simulink library "Library_SII_2018"  (R2018b)
settings: Solver=ode45  StartTime=0.0  StopTime=10.0  RelTol=1e-3  EnableMultiTasking=on
undefined symbols (not defined in the file or in its folder): coder, gcbh, r, simscape
libraries: fl_lib x157, nesl_utility x81, Library_SII2 x44, simulink x17, powerlib x12, mblibv1 x11, Simscape_SII_lib x11, elec_lib x10, Pneumatic_lib x4, $bdroot x2, peRmsMeasurement x1, powerlib_extras x1
(part 2 of 6)

== system Library_SII_2018/Mécanique ==
  Capteur de force FSR : Subsystem  mask(Capteur de force FSR){a=-0.8, b=5.2}
      mask help:
      | Modèle :
      | log(R) = a log(F) + b
      | avec :
      |   - F : force en N
      |   - R : résistance en Ohm
      mask DialogControl ParameterGroupVar Prompt: Paramètres
      mask Display: image('images/FSR.png')
  Capteur de puissance mécanique de rotation : Subsystem  mask(Capteur de puissance mécanique de rotation){}
      mask help:
      | Le bloc représente un capteur de puissance mécanique de rotation.
      | R et C sont des ports physiques conservatifs.
      |
      | P, T et W sont des ports Simulink délivrant les valeurs de :
      |  - la puissance mécanique traversant le bloc (en W)
      |  - le couple transmis à travers le bloc (en Nm)
      |  - la vitesse de rotation (en rad/s)
      |
      | Ces valeurs sont calculées par rapport au référentiel Ref.
      mask Display:
      | plot([149.600878633536;150.016472378793;150.47508104106;150.972287968219;151.50330478576;152.063017511447;152.646035805762;153.246744883819;153.859359588817;154.477980106257;155.096648782383;155.709407499646;156.310355056631;156.893703999851;157.453836360095;157.985357756531;158.483149347555;158.942417128023;159.358738098149;159.728102859405;160.046954227227;160.312221488639;160.521349974904;160.672325664379;160.763694578642;160.794576785101;160.764674871227;160.674276808796;160.524253180566;160.316048796087;160.051668777399;159.733659248606;159.365082815313;158.949489070056;158.490880407788;157.993673480629;157.462656663088;156.908284800231], [156.971389291536;157.430657072004;157.84697804213;158.216342803387;158.535194171208;158.80046143262;159.009589918885;159.16056560836;159.251934522623;159.282816729083;159.252914815208;159.162516752777;159.012493124547;158.804288740068;158.53990872138;158.221899192587;157.853322759294;157.437729014037;156.979120351769;156.48191342461;155.950896607069;155.391183881382;154.808165587067;154.20745650901;153.594841804012;152.976221286573;152.357552610446;151.744793893183;151.143846336199;150.560497392978;150.000365032735;149.468843636298;148.971052045274;148.511784264806;148.095463294681;147.726098533424;147.407247165603;147.144199990631])
      | plot([152.057635404444;152.93604260309;153.834625296826;154.744729643097;155.657590839533;156.564417533794;157.45647648909;158.325176690034;159.162152078811;159.959342124889;160.709069452336;161.404113777147;162.037781442523;162.603969882449;163.097226392739;163.512800643557;163.846690427691;164.095680203997;164.257372064819;164.330208829146;164.313489039122;164.27939575172], [142.228020686971;141.979030910664;141.817339049842;141.744502285515;141.761222075539;141.867337399197;142.061826307913;142.342815767178;142.707599694895;143.152665022428;143.673725527376;144.265763112236;144.923076131425;145.639334301243;146.40763966397;147.220593018964;148.070365181011;148.948772379657;149.847355073393;150.757459419663;151.6703206161;152.055850472277])
      | %plot([116.468514315784;116.438789536125;116.349901463023;116.202706137216;115.998621130155;115.739611892022;115.42817282337;115.067303252679;114.660478551187;114.211616663162;113.725040373958;113.205435679231;112.657806656235;112.087427271827;111.499790591278;110.900555877058;110.29549408704;109.690432297022;109.091197582803;108.503560902254;107.933181517846;107.38555249485;106.865947800123;106.379371510919;105.930509622894;105.523684921402;105.162815350711;104.851376282059;104.592367043926;104.388282036865;104.241086711057;104.152198637956;104.122473858297;104.152198637956;104.241086711057;104.388282036865;104.592367043926;104.851376282059;105.162815350711;105.523684921402;105.930509622894;106.379371510919;106.865947800123;107.38555249485;107.933181517846;108.503560902254;109.091197582803;109.690432297022;110.29549408704;110.900555877058;111.499790591278;112.087427271827;112.657806656235;113.205435679231;113.725040373958;114.211616663162;114.660478551187;115.067303252679;115.42817282337;115.739611892022;115.998621130155;116.202706137216;116.349901463023;116.438789536125;116.468514315784;116.468514315784], [111.618284136057;111.013222346039;110.413987631819;109.826350951271;109.255971566862;108.708342543866;108.188737849139;107.702161559936;107.253299671911;106.846474970419;106.485605399728;106.174166331075;105.915157092943;105.711072085881;105.563876760074;105.474988686973;105.445263907313;105.474988686973;105.563876760074;105.711072085881;105.915157092943;106.174166331075;106.485605399728;106.846474970419;107.253299671911;107.702161559936;108.188737849139;108.708342543866;109.255971566862;109.826350951271;110.413987631819;111.013222346039;111.618284136057;112.223345926075;112.822580640295;113.410217320843;113.980596705252;114.528225728247;115.047830422975;115.534406712178;115.983268600203;116.390093301695;116.750962872386;117.062401941038;117.321411179171;117.525496186232;117.67269151204;117.761579585141;117.7913043648;117.761579585141;117.67269151204;117.525496186232;117.321411179171;117.062401941038;116.750962872386;116.390093301695;115.983268600203;115.534406712178;115.047830422975;114.528225728247;113.980596705252;113.410217320843;112.822580640295;112.223345926075;111.618284136057;111.618284136057])
      | plot([239.23602886498;238.828071429858;237.608127977604;235.587947230552;232.78698463364;229.232214987837;224.957872668068;220.005121927465;214.421660463109;208.261260061133;201.583248745024;194.451939414329;186.936010476274;179.107844435155;171.042830809261;162.818640088593;154.514475725591;146.210311362589;137.986120641921;129.921107016027;122.092940974909;114.577012036853;107.445702706158;100.76769139005;94.607290988073;89.0238295237172;84.0710787831142;79.7967364633452;76.2419668175427;73.4410042206305;71.4208234735788;70.2008800213248;69.7929225862026;70.2008800213248;71.4208234735788;73.4410042206306;76.2419668175428;79.7967364633454;84.0710787831144;89.0238295237174;94.6072909880733;100.76769139005;107.445702706159;114.577012036853;122.092940974909;129.921107016027;137.986120641921;146.210311362589;154.514475725591;162.818640088593;171.042830809261;179.107844435155;186.936010476274;194.451939414329;201.583248745024;208.261260061133;214.421660463109;220.005121927465;224.957872668068;229.232214987837;232.78698463364;235.587947230552;237.608127977604;238.828071429858;239.23602886498;239.23602886498], [155.774275772274;147.47628550917;139.258209428443;131.199192095207;123.376846251889;115.866505365088;108.740498123116;102.067451871182;95.9116316925529;90.3323215006612;85.3832531026163;81.1120887325275;77.5599620381344;74.7610819412943;72.742403187363;71.5233667562631;71.1157126352191;71.5233667562631;72.742403187363;74.7610819412943;77.5599620381345;81.1120887325275;85.3832531026164;90.3323215006612;95.9116316925529;102.067451871182;108.740498123116;115.866505365089;123.376846251889;131.199192095207;139.258209428443;147.47628550917;155.774275772274;164.072266035377;172.290342116104;180.34935944934;188.171705292658;195.682046179459;202.808053421432;209.481099673365;215.636919851994;221.216230043886;226.165298441931;230.43646281202;233.988589506413;236.787469603253;238.806148357184;240.025184788284;240.432838909328;240.025184788284;238.806148357184;236.787469603253;233.988589506413;230.43646281202;226.165298441931;221.216230043886;215.636919851994;209.481099673365;202.808053421432;195.682046179459;188.171705292658;180.34935944934;172.290342116105;164.072266035378;155.774275772274;155.774275772274])
      | plot([252.715889364481;252.243022716633;250.828976737403;248.487369462568;245.240751850236;241.120390602797;236.165967051481;230.425195003451;223.953361231755;216.812793033479;209.072257983804;200.806301666664;192.094529760025;183.020841389688;173.672621134841;164.139897466795;154.514475725591;144.889053984387;135.356330316341;126.008110061494;116.934421691157;108.222649784518;99.9566934673787;92.2161584177032;85.075590219427;78.6037564477313;72.8629843997015;67.9085608483856;63.7881996009461;60.5415819886144;58.199974713779;56.7859287345493;56.3130620867014;56.7859287345493;58.1999747137791;60.5415819886146;63.7881996009463;67.9085608483858;72.8629843997018;78.6037564477315;85.0755902194273;92.2161584177035;99.9566934673791;108.222649784519;116.934421691157;126.008110061494;135.356330316341;144.889053984387;154.514475725591;164.139897466796;173.672621134841;183.020841389688;192.094529760025;200.806301666664;209.072257983803;216.812793033479;223.953361231755;230.425195003451;236.165967051481;241.120390602797;245.240751850236;248.487369462568;250.828976737403;252.243022716633;252.715889364481;252.715889364481], [154.514475725591;144.895228084285;135.36861905618;126.026395093992;116.958526921455;108.252343066071;99.9916888376535;92.2561188521535;85.1201308772245;78.6524483779929;72.9153586725213;67.9641130708855;63.8463947748555;60.6018596625959;58.2617543808809;56.8486154228053;56.3760520890355;56.8486154228053;58.2617543808809;60.6018596625959;63.8463947748555;67.9641130708856;72.9153586725213;78.652448377993;85.1201308772246;92.2561188521536;99.9916888376536;108.252343066072;116.958526921455;126.026395093992;135.36861905618;144.895228084285;154.514475725591;164.133723366898;173.660332395002;183.002556357191;192.070424529728;200.776608385111;209.037262613529;216.772832599029;223.908820573958;230.37650307319;236.113592778661;241.064838380297;245.182556676327;248.427091788587;250.767197070302;252.180336028377;252.652899362147;252.180336028377;250.767197070301;248.427091788587;245.182556676327;241.064838380297;236.113592778661;230.37650307319;223.908820573958;216.772832599029;209.037262613529;200.776608385111;192.070424529728;183.002556357191;173.660332395002;164.133723366898;154.514475725592;154.514475725591])
      | plot([154.514475725591;129.948374815285;179.017586633563;154.514475725591], [240.369848906994;203.583687543869;203.583687543869;240.369848906994])
      | %plot([105.382273904979;149.60125554353], [115.271704271436;156.971085816622])
      | plot([144.688035361469;144.688035361469], [152.057865634561;203.583687543869])
      | plot([164.277926087379;164.277926087379], [152.057865634561;203.583687543869])
      | plot([159.112745895982;159.616665914655], [149.60125554353;149.60125554353])
      | %plot([115.208714269102;159.364705905318], [107.901873998344;149.60125554353])
      | plot([0;311.800511553884;311.800511553884;0;0], [311.800511553884;311.800511553884;0;0;311.800511553884])
      | ;
      | color('red');
      | port_label('LConn', 1,'R')
      | port_label('RConn', 1,'C')
      | port_label('LConn', 2,'Ref')
      | port_label('output', 1,'P')
      | port_label('output', 2,'T')
      | port_label('output', 3,'W')
      | %port_label('RConn', 3,'A')
  Codeur incrémental : Subsystem  AncestorBlock=Library_SII/Signaux/Codeur incrémental  mask(Codeur incrémental bidirectionnel){p=1}
      mask prompts: p "Résolution du codeur [°]"
      mask help:
      | Codeur incrémental (linéaire ou rotatif)
      | En entrée : un signal analogique (quelle que soit la grandeur)
      | En sortie : deux signaux logiques de fréquence variable
      | Paramètre : pas du codeur (même grandeur que le signal d'entrée
      mask DialogControl ParameterGroupVar Prompt: Paramètre
      mask Display: image('codeur.png')
  Codeur incrémental v2 : Subsystem  AncestorBlock=Library_SII/Mécanique/Codeur incrémental  mask(Codeur incrémental bidirectionnel){p=1, U=5}
      mask prompts: p "Résolution du codeur [°]"; U "Amplitude des signaux"
      mask help:
      | Codeur incrémental (linéaire ou rotatif)
      | En entrée : un signal analogique (quelle que soit la grandeur)
      | En sortie : deux signaux logiques de fréquence variable
      | Paramètre : pas du codeur (même grandeur que le signal d'entrée
      mask DialogControl ParameterGroupVar Prompt: Paramètre
      mask Display: image('codeur.png')
  Corde : Subsystem  mask{L=0.2, S=1, E=210}
      mask prompts: L "Longueur [m]"; S "Section [mm²]"; E "Module d'élasticité [GPa]"
  Differentiel : Simscape_SII_lib/Differentiel  t_in_specify=off  t_in_priority=High  t_in=0 N*m  t_in_nominal_specify=off  t_in_nominal_unit=N*m  t_in_nominal_value=1  t_outG_specify=off  t_outG_priority=High  t_outG=0 N*m  t_outG_nominal_specify=off  t_outG_nominal_unit=N*m  t_outG_nominal_value=1  t_outD_specify=off  t_outD_priority=High  t_outD=0 N*m  t_outD_nominal_specify=off  t_outD_nominal_unit=N*m  t_outD_nominal_value=1
  Embrayage : Simscape_SII_lib/Embrayage  brkwy_trq=25 N*m  Col_trq=20 N*m  trans_coef=10 s/rad  vel_thr=1e-4 rad/s  w_specify=off  w_priority=High  w=0 rad/s  w_nominal_specify=off  w_nominal_unit=rad/s  w_nominal_value=1  t_specify=off  t_priority=High  t=0 N*m  t_nominal_specify=off  t_nominal_unit=N*m  t_nominal_value=1
  Embrayage SM : Subsystem  mask(Embrayage){axe=[0 0 1]}
      mask prompts: axe "Axe de la  liaison [x y z]"
      mask help:
      | Embrayage, basé sur une liaison pivot.
      |   C = Signal Simulink de commande
      |     C > 0 : état embrayé (transmission intégralle de la puissance)
      |     C = 0 : état débrayé (équivalent à une liaison pivot)
      |
      | Indiquer l'axe de la liaison par ses composantes dans World.
      mask Display:
      | image(imread('Mécanique/embrayage.png'))
      | port_label('lconn', 1, 'B')
      | port_label('rconn', 1, 'F')
      | port_label('input', 1, 'C')
  Engrenage droit SS : Subsystem  mask(Réducteur à engrenages droit){r=2, n=0.8, J=0.001}
      mask prompts: r "Rapport de transmission"; n "Rendement"; J "Inertie (kg/m^2)"
      mask help:
      | Réducteur à engrenages droit
      | P = Pignon
      | R = Roue
      | Ref = Référence
      |
      | Le rapport de réduction est défini par : wp/wr
      | Le rendement doit être compris entre 0.1 et 1
      mask Callback n:
      | ren = str2num(get_param(gcb,'n'));
      | if or((ren < 0.1),(ren > 1));
      |     errordlg('Le rendement doit etre compris entre 0.1 et 1','Erreur');
      | end;
      mask Display:
      | plot([0] , [0]);
      | 
      | color('red');
      | plot([30, 100] , [150, 150]);
      | plot([90, 110] , [180, 180]);
      | plot([90, 110] , [120, 120]);
      | plot([100, 100] , [120, 180]);
      | 
      | color('blue');
      | plot([100, 180] , [50, 50]);
      | plot([100, 100] , [0, 120]);
      | plot([90, 110] , [0, 0]);
      | 
      | color('black');
      | %image(imread('RoueVisSSFin.jpg'))
      | port_label('lconn', 1, 'P');
      | port_label('lconn', 2, 'Ref');
      | port_label('rconn', 1, 'R');
  Frein à courant de Foucault : Simscape_SII_lib/Frein à courant de Foucault  B=1 T  s=1 / 3.8e-8 S/m  e=3e-3 m  ra=20e-3 m  rd=120e-38 m  w_specify=off  w_priority=None  w=0 rad/s  w_nominal_specify=off  w_nominal_unit=rad/s  w_nominal_value=1  t_specify=off  t_priority=None  t=0 N*m  t_nominal_specify=off  t_nominal_unit=N*m  t_nominal_value=1
  Masse variable : Simscape_SII_lib/Masse variable  v_specify=off  v_priority=High  v=0 m/s  v_nominal_specify=off  v_nominal_unit=m/s  v_nominal_value=1  f_specify=off  f_priority=High  f=0 N  f_nominal_specify=off  f_nominal_unit=N  f_nominal_value=1
  Ressort lineaire (raideur variable) : Simscape_SII_lib/Ressort lineaire (raideur variable)  v_specify=off  v_priority=High  v=0 m/s  v_nominal_specify=off  v_nominal_unit=m/s  v_nominal_value=1  f_specify=off  f_priority=High  f=0 N  f_nominal_specify=off  f_nominal_unit=N  f_nominal_value=1  x_specify=off  x_priority=High  x=0 m  x_nominal_specify=off  x_nominal_unit=m  x_nominal_value=1
  Roue - Vis sans fin SS : Subsystem  mask(Engrenage à Roue et Vis sans fin){r=5, f=0.15, J=0.01, B=60}
      mask prompts: r "Rapport de transmission"; f "Coefficient de frottement"; J "Inertie (kg/m^2)"; B "Angle de denture  de la roue (°)"
      mask help:
      | Engrenage à Roue et Vis sans fin :
      | R = Roue
      | V = Vis
      | Ref = Référence
      |
      | Le rapport de transmission est défini par : r = Wv/Wr
      |
      | Les valeurs de l'angle de denture de la roue
      | et du coefficient de frottement
      | permettent de calculer le rendement (voir l'aide pour plus d'informations)
      | Selon que la vis ou la roue soit motrice, ce rendement varie
      | et l'on peut avoir irréversibilité.
      mask init:
      | % Angle de frottement (en rad)
      | P = atan(f);
      | 
      | % Angle de denture (en rad)
      | Br = pi*B/180;
      | 
      | % Rendements selon le sens
      | n1 = tan(Br)/tan(Br+P);
      | n2 = tan(Br-P)/tan(Br);
      mask Help:
      | Le rendement est calculé, selon le sens, par les expressions :
      |  - Vis motrice : n1 = tan(B)/tan(B+P)
      |  - Roue motrice : n2 = tan(B-P)/tan(B)
      | 
      | avec P = atan(f) : Angle de frottement
      mask Callback B:
      | if ( str2num(get_param(gcb, 'B')) <= 0);
      |      errordlg('L''angle de denture ne peut pas être négatif !','Erreur');
      | end;
      mask Display:
      | image(imread('Mécanique/RoueVisSSFin.jpg'));
      | port_label('lconn', 1, 'V');
      | port_label('lconn', 2, 'Ref');
      | port_label('rconn', 1, 'R');
  Roue libre SM : Subsystem  mask(Roue libre){axe=[1 0 0], kv=0.01}
      mask prompts: axe "Vecteur directeur [x y z]"; kv "Coefficient de frottement visqueux (Nm/(rad/s))"
      mask help:
      | Roue libre, basée sur une liaison pivot, mais la rotation n'est possible
      | que dans un seul sens.
      | Pour inverser le sens, inverser les connections B et F.
      |
      | Indiquer l'axe de la liaison par ses composantes dans World.
      mask Display:
      | image(imread('Mécanique/Roue_libre.png'))
      | port_label('lconn', 1, 'B')
      | port_label('rconn', 1, 'F')
  Réducteur avec rendement : Simscape_SII_lib/Réducteur avec rendement  rapport_transmission=10  rendement=0.8  t_in_specify=off  t_in_priority=High  t_in=0 N*m  t_in_nominal_specify=off  t_in_nominal_unit=N*m  t_in_nominal_value=1  t_out_specify=off  t_out_priority=High  t_out=0 N*m  t_out_nominal_specify=off  t_out_nominal_unit=N*m  t_out_nominal_value=1
  Réducteur avec rendement et frottement : Simscape_SII_lib/Réducteur avec rendement et frottement  rapport_transmission=10  rendement=0.8  Col_trq=1 N*m  t_in_specify=off  t_in_priority=None  t_in=0 N*m  t_in_nominal_specify=off  t_in_nominal_unit=N*m  t_in_nominal_value=1  t_out_specify=off  t_out_priority=None  t_out=0 N*m  t_out_nominal_specify=off  t_out_nominal_unit=N*m  t_out_nominal_value=1
  Train epicycloidal : Simscape_SII_lib/Train epicycloidal  ratio=2  t_R_specify=off  t_R_priority=High  t_R=0 N*m  t_R_nominal_specify=off  t_R_nominal_unit=N*m  t_R_nominal_value=1  t_S_specify=off  t_S_priority=High  t_S=0 N*m  t_S_nominal_specify=off  t_S_nominal_unit=N*m  t_S_nominal_value=1  t_C_specify=off  t_C_priority=High  t_C=0 N*m  t_C_nominal_specify=off  t_C_nominal_unit=N*m  t_C_nominal_value=1

== system Library_SII_2018/Signaux ==
  Codeur incrémental : Subsystem  mask(Codeur incrémental bidirectionnel){p=r}
      mask prompts: p "Pas du codeur"
      mask help:
      | Codeur incrémental (linéaire ou rotatif)
      | En entrée : un signal analogique (quelle que soit la grandeur)
      | En sortie : deux signaux logiques de fréquence variable
      | Paramètre : pas du codeur (même grandeur que le signal d'entrée
      mask DialogControl ParameterGroupVar Prompt: Paramètre
      mask Display: image('codeur.svg')
  Contrôle de régime : Subsystem  mask(Controleur de régime){vl=0.8, al=1}
      mask prompts: vl "Vitesse limite (1/s)"; al "Accélération limite (1/s²)"
      mask help:
      | Permet de limiter la vitesse et l'accélération de variation d'un signal
      | à partir d'un échelon.
      mask Callback al:
      | if str2num(get_param(gcb, 'vl'))<=0
      | 	error('La vitesse limite doit être strictement positive !')
      | end
      | if str2num(get_param(gcb, 'al'))<=0
      | 	error('L''accélération limite doit être strictement positive')
      | end
      mask Display:
      | color('red');
      | x = [10 15 20 25 30 35 40 45 55 60 65 70 75 80 85 90];
      | y = [10 10.68 12.72 16.12 20.88 27 34.48 41.96 58.04 65.52 73 79.12 83.88 87.28 89.32 90];
      | plot(x/100, y/100);
      | plot(x/100, (y-1)/100);
      | plot(x/100, (y+1)/100);
  Frequence-Metre : Subsystem  mask(Fréquence-mètre){Ts=100e-6, Fs=6, spec=on, plage=[-1 -1]}
      mask prompts: Ts "Pèriode d'échantillonage (s)"; Fs "Fréquence de mesure (Hz)"; spec "Tracer un spectrogramme"; plage "Plage de fréquence du spectrogramme (-1 = auto)"
      mask help:
      | Estimation de la fréquence principale d'un signal.
      | - Période d'echantillonage : période en secondes entre deux échantillons
      | du signal. Le solveur doit être réglé en mode "Fixed-step" et cette période
      | doit être égale au paramètre "Fixed-step size".
      |
      | - Fréquence de mesure : fréquence entre deux mesures du fréquence-mètre en Hertz.
      |
      | La mesure est soumise à un compromis temps de calcul/précision.
      | Pour augmenter la précision, diminuer la période d'échantillonage
      | et choisir une fréquence de mesure au moins 10 fois inférieure à la fréquence
      | à mesurer.
      |
      | Pour afficher un spectrogramme, cocher la case "Tracer un spectrogramme"
      | et renseigner la plage de fréquence ([-1 -1] = auto)
      mask init:
      | N=fix((1/Fs)/Ts);
      mask Callback spec:
      | dd = get_param(gcb,'spec');
      | if strcmp(dd,'on'),
      |     set_param(gcb,'MaskEnables',{'on';'on';'on';'on'}),
      | else
      |     set_param(gcb,'MaskEnables',{'on';'on';'on';'off'}),
      | end
  Générateur de signal carré : Subsystem  mask(Générateur de signal carré){t=16, a=1, d=5}
      mask prompts: t "Retard (s)"; a "Amplitude"; d "Durée (s)"
      mask help:
      | Signal "carré" unique, à amplitude, durée et retard contrôlés.
      | Paramètres :
      |   Retard (s)
      |   Amplitude
      |   Durée (s)
      mask Display:
      | %origine
      | ox = 10;
      | oy = 10;
      | 
      | %fleche
      | l = 10;
      | e = 5;
      | 
      | %dimension
      | x = 300;
      | y = 200;
      | 
      | % ecarts
      | dx = 30;
      | dy = 30;
      | 
      | h = y-4*l;
      | 
      | %axes
      | color('black');
      | plot([dx;dx;x], [y;dy;dy])
      | plot([dx-e;dx;dx+e], [y-2*e;y;y-2*e])
      | plot([x-l;x;x-l], [dy-e;dy;dy+e])
      | plot([0], [0])
      | 
      | %textes
      | text(x/3,15, 't0')
      | text(dx,15, '0')
      | text(15,h, 'a')
      | text(x/2,h/2, 'd')
      | 
      | %courbe
      | color('red');
      | plot([dx;x/3;x/3;2*x/3;2*x/3;x-2*l], [dy; dy;h;h;dy;dy])
  Générateur de signal pas : Subsystem  mask(Générateur de signal carré){t=0.5, a=10, p=5}
      mask prompts: t "Retard (s)"; a "Amplitude"; p "Pente"
      mask help:
      | Signal "carré" unique, à amplitude, durée et retard contrôlés.
      | Paramètres :
      |   Retard (s)
      |   Amplitude
      |   Durée (s)
      mask Display:
      | %origine
      | ox = 10;
      | oy = 10;
      | 
      | %fleche
      | l = 10;
      | e = 5;
      | 
      | %dimension
      | x = 300;
      | y = 200;
      | 
      | % ecarts
      | dx = 30;
      | dy = 30;
      | 
      | h = y-4*l;
      | 
      | %axes
      | color('black');
      | plot([dx;dx;x], [y;dy;dy])
      | plot([dx-e;dx;dx+e], [y-2*e;y;y-2*e])
      | plot([x-l;x;x-l], [dy-e;dy;dy+e])
      | plot([0], [0])
      | 
      | %textes
      | text(x/3,15, 't0')
      | text(dx,15, '0')
      | text(15,h, 'a')
      | text(x/2,h/2, 'p')
      | 
      | %courbe
      | color('red');
      | plot([dx; x/3; 2*x/3; x-2*l], [dy; dy; h; h])
      | 
      | %image(imread('carre.jpg'))
  Générateur de signal périodique carré : Subsystem  mask(Générateur de signal logique périodique){}
      mask help:
      | Générateur de signal logique de fréquence variable.
      |
      | En entrée :
      |  * la valeur de la fréquence (en Hz)
      |  * le rapport cyclique (valeur entre 0 et 1)
      |
      | En sortie : un signal logique (entre 0 et 1)
      mask Display: image('carre.svg')
  PS Saturation variable : SimscapeBlock  AncestorBlock=Simscape_SII_lib/PS Saturation  DialogController=NetworkEngine.DynNeDlgSource  LoadFcn=simscape.compiler.sli.internal.callback('LoadFcn',gcbh);  SourceFile=Simscape_SII.saturation_var  mask(PS Saturation){ComponentPath=Simscape_SII.saturation_var, ComponentVariants=Simscape_SII.saturation_var, ComponentVariantNames=saturation, ClassName=saturation, SchemaVersion=1}
      mask help:
      | This block imposes upper and lower bounds on the output signal. When the input signal is within the range specified by the Lower limit and Upper limit parameters, the input signal passes through unchanged. When the input signal is outside these bounds, the signal is clipped to the upper or lower bound.
      |
      | Both the input and the output are physical signal ports.
      mask init:
      | simscape.compiler.sli.internal.preinitmask(gcb);
      settings: CopyFcn=simscape.compiler.sli.internal.callback('CopyFcn',gcbh);  DeleteFcn=simscape.compiler.sli.internal.callback('DeleteFcn',gcbh);  ModelCloseFcn=simscape.compiler.sli.internal.callback('ModelCloseFcn',gcbh);  PreSaveFcn=simscape.compiler.sli.internal.callback('PreSaveFcn',gcbh);  PostSaveFcn=simscape.compiler.sli.internal.callback('PostSaveFcn',gcbh);  PreCopyFcn=simscape.compiler.sli.internal.callback('PreCopyFcn',gcbh);  PreDeleteFcn=simscape.compiler.sli.internal.callback('PreDeleteFcn',gcbh);
      mask Help: web(nesl_help(gcbh))
      mask Display:
      | plot([0.15 0.85],[.5 .5],[.5 .5],[0.05 0.95],0.15+0.7*[0 .25 .75 1],0.05+0.9*[.25 .25 .75 .75]);
      | disp('        L\n\n\n')
      | disp('\n\n\n\n-L           ');
      | color('red');
      | port_label('RConn', 1,'S');
      | port_label('LConn', 2,'L');
      | port_label('LConn', 1,'E');
  Signal carré périodique symétrique : Subsystem  mask{T=20e-3, a=10, r=50}
      mask prompts: T "Période [s]"; a "Amplitude (+-)"; r "Rapport cyclique [%]"
      mask Display:
      | %origine
      | ox = 10;
      | oy = 10;
      | 
      | %fleche
      | l = 10;
      | e = 5;
      | 
      | %dimension
      | x = 300;
      | y = 200;
      | 
      | % ecarts
      | dx = 40;
      | dy = 30;
      | 
      | h = y-4*l;
      | 
      | %axes
      | color('black');
      | plot([dx;dx], [y;dy])
      | plot([dx;x], [y/2;y/2])
      | 
      | plot([dx-e;dx;dx+e], [y-2*e;y;y-2*e])
      | plot([x-l;x;x-l], [dy-e;dy;dy+e])
      | plot([0], [0])
      | 
      | %textes
      | %text(x/3,15, 't0')
      | text(dx/2,y/2, '0')
      | text(dx/2,h, 'a')
      | text(dx/2,dy, '-a')
      | %text(x/2,h/2, 'd')
      | 
      | %courbe
      | color('red');
      | plot([dx;x/3;x/3;2*x/3;2*x/3;x-2*l], [dy; dy;h;h;dy;dy])
  Tracé XY point à point : MATLAB Function  InitFcn=titre = get_param(gcb, 'titre');  TreatAsAtomicUnit=on  SystemSampleTime=0.2  mask(Tracé XY point à point){titre=0, style=-o, echellex=linéaire, autox=on, xmin=-1, xmax=0, echelley=linéaire, autoy=on, ymin=2, ymax=3}
      mask prompts: echellex "Échelle"; autox "Automatique"; echelley "Échelle"; autoy "Automatique"
      mask help:
      | Bloc permettant d'afficher une fenêtre de tracé XY
      |
      | Conseils d'utilisation en mode "temps réel" :
      |  - mettre le temps de simulation à inf
      |  - utiliser le bloc Real-Time Pacer
      |  - réduire la période d'échantillonnage du bloc de tracé (clic-droit+Bloc Parameters)
      |   de manière à obtenir 5 à 10 points par secondes
      |      exemple : Real-Time Pacer/Speedup = 1  --> Tracé XY/Sample time = 0.2
      |  - utiliser un solveur de type Variable Step, type Automatique
      mask init:
      | fh = findobj( 'Type', 'Figure', 'Name', titre);
      | if length(fh) > 0 % il y a déja une figure qui porte le nom titre
      |     f = fh(1);
      |     figure(f);
      | else
      |     f = figure('Name',titre);
      | end
      | 
      | clf;
      | hold on;
      | set(gca,'XLim',[xmin xmax],'Ylim',[ymin ymax]);
      | plot([],[], style,'Markersize',6,'MarkerFaceColor','g');
      | if autox
      |     if autoy
      |         axis 'auto xy'
      |     else
      |         axis 'auto x'
      |     end
      | else
      |     if autoy
      |         axis 'auto y'
      |     else
      |         axis 'manual'
      |     end
      | end
      | 
      | if echellex == 1
      |     set(gca, 'XScale', 'lin');
      | else
      |     set(gca, 'XScale', 'log');
      | end
      | 
      | if echelley == 1
      |     set(gca, 'YScale', 'lin');
      | else
      |     set(gca, 'YScale', 'log');
      | end
  Trapèze : Subsystem  mask{a=1, t0=0, p=0.2, th=4}
      mask prompts: a "Amplitude"; t0 "Instant début (s)"; p "Pente"; th "Temps haut (s)"
      mask Display:
      | %origine
      | ox = 10;
      | oy = 10;
      | 
      | %fleche
      | l = 10;
      | e = 5;
      | 
      | %dimension
      | x = 300;
      | y = 200;
      | 
      | % ecarts
      | dx = 30;
      | dy = 30;
      | 
      | h = y-4*l;
      | 
      | %axes
      | color('black');
      | plot([dx;dx;x], [y;dy;dy])
      | plot([dx-e;dx;dx+e], [y-2*e;y;y-2*e])
      | plot([x-l;x;x-l], [dy-e;dy;dy+e])
      | plot([0], [0])
      | 
      | %textes
      | text(x/3,15, 't0')
      | text(dx,15, '0')
      | text(15,h, 'a')
      | text(x/2,h/2, 'p')
      | 
      | %courbe
      | color('red');
      | plot([dx; x/5; 2*x/5; 3*x/5; 4*x/5; x-2*l], [dy; dy; h; h; dy; dy])
      | 
      | 
      | %image(imread('carre.jpg'))
  bascule : Stateflow chart  TreatAsAtomicUnit=on
  bascule 2 sorties : Stateflow chart  TreatAsAtomicUnit=on

== system Library_SII_2018/ThermLiquid ==
  Capteur Pression Température [bar] et [°C] : Subsystem  mask(Capteur de Pression et de Température (TL)){}
      mask help:
      | Capteur de Pression et de Température.
      | Pression absolue en bar
      | Température absolue en °C
  Vase d'expansion : Subsystem  mask{V=20, p0=4, T0=20}
      mask prompts: V "Volume [L]"; p0 "Pression initiale [bar]"; T0 "Température initiale [°C]"
      mask Display: image('ThermLiquid/vase_expansion.jpg')

== system Library_SII_2018/Thermique ==
  Capteur température : Subsystem  mask(Capteur de température){}
      mask help: Température absolue en °C
  Incidence surface : Subsystem  mask{lat=[45 46 46], lon=[-3 05 10], T_air=20, Hr=0.5, P_Atm=98232, B=0.1}
      mask prompts: lat "Latitude [°, ', '']"; lon "Longitude [°, ', '']"; T_air "Température de l'air (°C)"; Hr "Humidité relative"; P_Atm "Pression atmosphérique (Pa)"; B "Coefficient de trouble atmosphérique"
      mask help:
      | Coefficient de trouble atmosphérique
      | B = 0,02 pour un lieu situé en montagne
      | B = 0,05 pour un lieu rural
      | B = 0,10 pour un lieu urbain
      | B = 0,20 pour un lieu industriel (atmosphère polluée)
      mask Display:
      | [rgb, map, alpha] = imread('incidence.png', 'png');
      | image(rgb, [0.3, 0.05, 0.55, 0.7]);
      | port_label('input', 1, 'Energie soleil [W/m²]');
      | port_label('input', 3, 'Azimut soleil [°]');
      | port_label('input', 2, 'Hauteur soleil [°]');
      | port_label('input', 4, 'orientation surface [Nord = 0°]');
      | port_label('input', 5, 'inclinaison surface [Horiz = 0°]');
      | port_label('output', 1, 'Energie reçue [W/m²]');
  Paroi : Subsystem  mask(Paroi){m=Béton, d=off, lambda=0.92, c=880, mv=2200, s=1, e=10, Ti=20}
      mask prompts: m "Matériau"; d "Utiliser des valeurs personnalisées"; lambda "Conductivité thermique (W.m<sup>-1</sup>.K<sup>-1</sup>)"; c "Capacité thermique (J.kg<sup>-1</sup>.K<sup>-1</sup>)"; mv "Masse volumique (kg/m<sup>3</sup>)"; s "Surface de la paroi (m<sup>2</sup>)"; e "Epaisseur de la paroi (cm)"; Ti "Température initiale (°C)"
      mask help:
      | Modèle d'une paroi opaque (transmission de la chaleur par conduction).
      |
      | 1) Choisir un matériau
      | ou bien indiquer les caractéristiques thermiques d'un matériau
      | - Conductivité thermique (W.m-1.K-1)
      | - Capacité thermique (J.kg-1.K-1)
      | - Masse volumique (kg/m3)
      |
      | 2) Indiquer les dimensions de la paroi :
      | - Surface (m²)
      | - Epaisseur (cm)
      |
      | 3) Préciser la température initiale (°C)
      |
      | ==> Sortie :
      | T = Température au coeur de la paroi (°C)
      mask init:
      | % Conversion de la température
      | Ti = 273.15+Ti;
      | 
      | % Calcul de la masse
      | masse = mv * s * e / 100;
      | 
      | CaractMateriaux;
      mask Help:
      | Modèle d'une paroi opaque (transmission de la chaleur par conduction).
      | 
      | 1) Choisir un matériau
      | ou bien indiquer les caractéristiques thermiques d'un matériau
      | - Conductivité thermique (W.m<sup>-1</sup>.K<sup>-1</sup>)
      | - Capacité thermique (J.kg<sup>-1</sup>.K<sup>-1</sup>)
      | - Masse volumique (kg/m<sup>3</sup>)
      | 
      | 2) Indiquer les dimensions de la paroi :
      | - Surface (m²)
      | - Epaisseur (cm)
      | 
      | 3) Préciser la température initiale (°C)
      | 
      | ==> Sortie :
      | T = Température au coeur de la paroi (°C)
      | 
      | 
      | Il est possible de trouver les caractéristiques thermiques des principaux
      | matériaux de construction sur le site :
      | <a href="http://www.maison.com/architecture/maison-basse-consommation/quoi-construire-murs-maison-4881/"><tt>www.maison.com</tt></a>
      mask TypeOptions m: Shiste ardoise | Brique pleine | Béton | Béton armé | Béton cellulaire | Brique terre cuite pleine | Parpaing | Laine de verre | Laine de roche | Verre | Parpaing Monomur | PVC | Roche volcanique | Sapin | Panneau de particules agglomérées | Platre
      mask Callback m:
      | CaractMateriaux;
      | dd = get_param(gcb,'d');
      | if strcmp(dd,'off');
      |     mm =  get_param(gcb, 'm');
      |     set_param(gcb, 'lambda',Materiau(mm).Conductivite);
      |     set_param(gcb, 'mv',Materiau(mm).MasseVol);
      |     set_param(gcb, 'c',Materiau(mm).Capacite);
      | end
      mask Callback d:
      | maskStr = get_param(gcb,'MaskValues');
      | dd = get_param(gcb,'d');
      | if strcmp(dd,'on');
      |     set_param(gcb,'MaskEnables',{'on';'on';'on';'on';'on';'on';'on';'on'}),
      | else
      |     set_param(gcb,'MaskEnables',{'on';'on';'off';'off';'off';'on';'on';'on'}),
      | end
      mask DialogControl ParameterTabVar0 Prompt: Matériau
      mask DialogControl ParameterTabVar01 Prompt: Dimensions
      mask DialogControl ParameterTabVar012 Prompt: Conditions initiales
      mask Display:
      | image(imread(['Thermique/' Materiau(get_param(gcb, 'm')).Image]), [0.2, 0, 0.6, 0.85]);
      | port_label('lconn', 1, 'G');
      | port_label('rconn', 1, 'D');
      | port_label('output', 1, 'T');
      | 
      | 
      | text(0.5,0.95, get_param(gcb, 'm'), ...
      |      'HorizontalAlignment','center');
  Paroi (avec  rayonnement) : Subsystem  mask(Paroi){m=Parpaing, d=off, lambda=0.952, c=1080, mv=1185, s=200, e=10, Ti=20, Conv_Int=25, Conv_Ext=35}
      mask prompts: m "Matériau"; d "Utiliser des valeurs personnalisées"; lambda "Conductivité thermique (W.m<sup>-1</sup>.K<sup>-1</sup>)"; c "Capacité thermique (J.kg<sup>-1</sup>.K<sup>-1</sup>)"; mv "Masse volumique (kg/m<sup>3</sup>)"; s "Surface de la paroi (m<sup>2</sup>)"; e "Epaisseur de la paroi (cm)"; Ti "Température initiale (°C)"; Conv_Int "Coefficient de convection Intérieur (W/m²/K)"; Conv_Ext "Coefficient de convection Extérieur (W/m²/K)"
      mask help:
      | Modèle d'une paroi opaque. Transmission de la chaleur par :
      |  * conduction,
      |  * convection,
      |  * et rayonnement grace au port C.
      |
      | 1) Choisir un matériau
      | ou bien indiquer les caractéristiques thermiques d'un matériau
      | - Conductivité thermique [W.m-1.K-1]
      | - Capacité thermique [J.kg-1.K-1]
      | - Masse volumique [kg/m3]
      |
      | 2) Indiquer les dimensions de la paroi :
      | - Surface [m²]
      | - Epaisseur [cm]
      |
      | 3) Préciser la température initiale [°C]
      |
      | ==> Sortie :
      | T = Température au coeur de la paroi [°C]
      | F = Flux de chaleur traversant la paroi [W]
      mask init:
      | % Conversion de la température
      | Ti = 273.15+Ti;
      | 
      | % Calcul de la masse
      | masse = mv * s * e / 100;
      | 
      | CaractMateriaux;
      mask Help:
      | Modèle d'une paroi opaque (transmission de la chaleur par conduction).
      | 
      | 1) Choisir un matériau
      | ou bien indiquer les caractéristiques thermiques d'un matériau
      | - Conductivité thermique (W.m<sup>-1</sup>.K<sup>-1</sup>)
      | - Capacité thermique (J.kg<sup>-1</sup>.K<sup>-1</sup>)
      | - Masse volumique (kg/m<sup>3</sup>)
      | 
      | 2) Indiquer les dimensions de la paroi :
      | - Surface (m²)
      | - Epaisseur (cm)
      | 
      | 3) Préciser la température initiale (°C)
      | 
      | ==> Sortie :
      | T = Température au coeur de la paroi (°C)
      | 
      | 
      | Il est possible de trouver les caractéristiques thermiques des principaux
      | matériaux de construction sur le site :
      | <a href="http://www.maison.com/architecture/maison-basse-consommation/quoi-construire-murs-maison-4881/"><tt>www.maison.com</tt></a>
      mask TypeOptions m: Shiste ardoise | Brique pleine | Béton | Béton armé | Béton cellulaire | Brique terre cuite pleine | Parpaing | Laine de verre | Laine de roche | Verre | Parpaing Monomur | PVC | Roche volcanique | Sapin | Panneau de particules agglomérées | Platre
      mask Callback m:
      | CaractMateriaux;
      | dd = get_param(gcb,'d');
      | if strcmp(dd,'off');
      |     mm =  get_param(gcb, 'm');
      |     set_param(gcb, 'lambda',Materiau(mm).Conductivite);
      |     set_param(gcb, 'mv',Materiau(mm).MasseVol);
      |     set_param(gcb, 'c',Materiau(mm).Capacite);
      | end
      mask Callback d:
      | maskStr = get_param(gcb,'MaskValues');
      | dd = get_param(gcb,'d');
      | if strcmp(dd,'on');
      |     set_param(gcb,'MaskEnables',{'on';'on';'on';'on';'on';'on';'on';'on';'on';'on'}),
      | else
      |     set_param(gcb,'MaskEnables',{'on';'on';'off';'off';'off';'on';'on';'on';'on';'on'}),
      | end
      mask DialogControl ParameterTabVar0 Prompt: Matériau
      mask DialogControl ParameterTabVar01 Prompt: Dimensions
      mask DialogControl ParameterTabVar012 Prompt: Conditions initiales
      mask DialogControl ParameterTabVar0123 Prompt: Convection
      mask Display:
      | image(imread(['Thermique/' Materiau(get_param(gcb, 'm')).Image]), [0.2, 0, 0.6, 0.85]);
      | port_label('lconn', 1, 'Int');
      | port_label('rconn', 1, 'Ext');
      | port_label('rconn', 2, 'Ray');
      | port_label('output', 1, 'T');
      | port_label('output', 2, 'Fext');
      | port_label('output', 3, 'Fint');
      | 
      | 
      | text(0.5,0.95, get_param(gcb, 'm'), ...
      |      'HorizontalAlignment','center');
  Paroi (avec convection) : Subsystem  mask(Paroi){m=Parpaing, d=off, lambda=0.952, c=1080, mv=1185, s=200, e=10, Ti=20, Conv_Int=25, Conv_Ext=35}
      mask prompts: m "Matériau"; d "Utiliser des valeurs personnalisées"; lambda "Conductivité thermique (W.m<sup>-1</sup>.K<sup>-1</sup>)"; c "Capacité thermique (J.kg<sup>-1</sup>.K<sup>-1</sup>)"; mv "Masse volumique (kg/m<sup>3</sup>)"; s "Surface de la paroi (m<sup>2</sup>)"; e "Epaisseur de la paroi (cm)"; Ti "Température initiale (°C)"; Conv_Int "Coefficient de convection Intérieur (W/m²/K)"; Conv_Ext "Coefficient de convection Extérieur (W/m²/K)"
      mask help:
      | Modèle d'une paroi opaque. Transmission de la chaleur par :
      |  * conduction,
      |  * convection,
      |  * et rayonnement grace au port C.
      |
      | 1) Choisir un matériau
      | ou bien indiquer les caractéristiques thermiques d'un matériau
      | - Conductivité thermique [W.m-1.K-1]
      | - Capacité thermique [J.kg-1.K-1]
      | - Masse volumique [kg/m3]
      |
      | 2) Indiquer les dimensions de la paroi :
      | - Surface [m²]
      | - Epaisseur [cm]
      |
      | 3) Préciser la température initiale [°C]
      |
      | ==> Sortie :
      | T = Température au coeur de la paroi [°C]
      | F = Flux de chaleur traversant la paroi [W]
      mask init:
      | % Conversion de la température
      | Ti = 273.15+Ti;
      | 
      | % Calcul de la masse
      | masse = mv * s * e / 100;
      | 
      | CaractMateriaux;
      mask Help:
      | Modèle d'une paroi opaque (transmission de la chaleur par conduction).
      | 
      | 1) Choisir un matériau
      | ou bien indiquer les caractéristiques thermiques d'un matériau
      | - Conductivité thermique (W.m<sup>-1</sup>.K<sup>-1</sup>)
      | - Capacité thermique (J.kg<sup>-1</sup>.K<sup>-1</sup>)
      | - Masse volumique (kg/m<sup>3</sup>)
      | 
      | 2) Indiquer les dimensions de la paroi :
      | - Surface (m²)
      | - Epaisseur (cm)
      | 
      | 3) Préciser la température initiale (°C)
      | 
      | ==> Sortie :
      | T = Température au coeur de la paroi (°C)
      | 
      | 
      | Il est possible de trouver les caractéristiques thermiques des principaux
      | matériaux de construction sur le site :
      | <a href="http://www.maison.com/architecture/maison-basse-consommation/quoi-construire-murs-maison-4881/"><tt>www.maison.com</tt></a>
      mask TypeOptions m: Shiste ardoise | Brique pleine | Béton | Béton armé | Béton cellulaire | Brique terre cuite pleine | Parpaing | Laine de verre | Laine de roche | Verre | Parpaing Monomur | PVC | Roche volcanique | Sapin | Panneau de particules agglomérées | Platre
      mask Callback m:
      | CaractMateriaux;
      | dd = get_param(gcb,'d');
      | if strcmp(dd,'off');
      |     mm =  get_param(gcb, 'm');
      |     set_param(gcb, 'lambda',Materiau(mm).Conductivite);
      |     set_param(gcb, 'mv',Materiau(mm).MasseVol);
      |     set_param(gcb, 'c',Materiau(mm).Capacite);
      | end
      mask Callback d:
      | maskStr = get_param(gcb,'MaskValues');
      | dd = get_param(gcb,'d');
      | if strcmp(dd,'on');
      |     set_param(gcb,'MaskEnables',{'on';'on';'on';'on';'on';'on';'on';'on';'on';'on'}),
      | else
      |     set_param(gcb,'MaskEnables',{'on';'on';'off';'off';'off';'on';'on';'on';'on';'on'}),
      | end
      mask DialogControl ParameterTabVar0 Prompt: Matériau
      mask DialogControl ParameterTabVar01 Prompt: Dimensions
      mask DialogControl ParameterTabVar012 Prompt: Conditions initiales
      mask DialogControl ParameterTabVar0123 Prompt: Convection
      mask Display:
      | image(imread(['Thermique/' Materiau(get_param(gcb, 'm')).Image]), [0.2, 0, 0.6, 0.85]);
      | port_label('lconn', 1, 'Int');
      | port_label('rconn', 1, 'Ext');
      | port_label('rconn', 2, 'Ray');
      | port_label('output', 1, 'T');
      | port_label('output', 2, 'Fext');
      | port_label('output', 3, 'Fint');
      | 
      | 
      | text(0.5,0.95, get_param(gcb, 'm'), ...
      |      'HorizontalAlignment','center');
  Rayonnement solaire : Subsystem  mask{lat=[45 46 46], lon=[-3 05 10], T_air=20, Hr=0.5, P_Atm=98232, B=0.1}
      mask prompts: lat "Latitude [°, ', '']"; lon "Longitude [°, ', '']"; T_air "Température de l'air (°C)"; Hr "Humidité relative"; P_Atm "Pression atmosphérique (Pa)"; B "Coefficient de trouble atmosphérique"
      mask help:
      | Coefficient de trouble atmosphérique
      | B = 0,02 pour un lieu situé en montagne
      | B = 0,05 pour un lieu rural
      | B = 0,10 pour un lieu urbain
      | B = 0,20 pour un lieu industriel (atmosphère polluée)
      mask Display:
      | [rgb, map, alpha] = imread('Soleil.png', 'png');
      | image(rgb, [0.3, 0.1, 0.4, 0.8]);
      | port_label('input', 1, 'jour (1er janvier = 1)');
      | port_label('input', 2, 'heure [s] (minuit = 0s)');
      | port_label('output', 1, 'Energie soleil [W/m²]');
      | port_label('output', 3, 'Azimut soleil [°]');
      | port_label('output', 2, 'Hauteur soleil [°]');
  Variable convective Heat Transfer : Simscape_SII_lib/Variable convective Heat Transfer  area=1e-4 m^2  T_specify=off  T_priority=High  T=0 K  T_nominal_specify=off  T_nominal_unit=K  T_nominal_value=1  Q_specify=off  Q_priority=High  Q=0 J/s  Q_nominal_specify=off  Q_nominal_unit=W  Q_nominal_value=1
  Vitrage : Subsystem  mask(Vitrage){typ=Simple, gaz=Air, itr=off, s=1, ev=4, evi=3.3, eg=6, egi=10, ev0=6, ege=10, eve=3.3, R=0.17181, U=5.8203, Ti=20}
      mask prompts: typ "Type de vitrage"; gaz "Type de gaz"; itr "Couche ITR"; s "Surface de la paroi (m<sup>2</sup>)"; ev "Epaisseur du verre (mm)"; evi "Epaisseur du verre intérieur (mm)"; eg "Epaisseur de la lame de gaz (mm)"; egi "Epaisseur de la lame de gaz coté intérieur (mm)"; ev0 "Epaisseur du verre intermédiaire (mm)"; ege "Epaisseur de la lame de gaz coté extérieur (mm)"; eve "Epaisseur du verre extérieur (mm)"; R "Résistance thermique (m².K/W)"; U "Coefficient thermique Ug (W/(m².K))"; Ti "Température initiale (°C)"
      mask help:
      | Modèle d'une vitre de fenêtre verticale.
      |
      | Type de vitrage : "Simple", "Double" ou "Triple"
      | Type de Gaz : le gaz remplissant les intervalles entre les parois de verre
      | Couche ITR = Isolation Thermique Renforcée : verre revêtu d'une couche
      | transparente d'oxydes métalliques nobles ou d'argent permettant
      | de retenir la chaleur à l'intérieur du logement.
      |
      | Ti et Te sont les températures de surfaces intérieure et extérieure.
      |
      | Résistance thermique et Coefficient Ug : ils caractérisent les transferts
      | thermiques à travers une paroi par conduction, convection et rayonnement.
      | L’ensemble de ces transferts thermiques est défini, selon la norme EN 673,
      | pour une vitesse de vent, des émissivités et des températures normalement
      | rencontrées dans le domaine du bâtiment.
      | (voir le document tarcog mathematical model.pdf pour plus de détails)
      mask init:
      | % Conversion de la température
      | %Ti = 273.15+Ti;
      | CaractMateriaux;
      | 
      | infini = '1e12';
      | sgaz = get_param(gcb, 'gaz');
      | sitr = get_param(gcb, 'itr');
      | switch typ
      |     case 1
      |         set_param([gcb '/Verre_int'], 'lambda', '1.2')
      |         set_param([gcb '/Verre_int'], 'e', num2str(ev))
      |         set_param([gcb '/Verre'], 'lambda', infini)
      |         set_param([gcb '/Verre_ext'], 'lambda', infini)
      |         set_param([gcb '/Gaz_int'], 'heat_tr_coeff', infini)
      |         set_param([gcb '/Gaz_ext'], 'heat_tr_coeff', infini)
      |    
      |     case 2
      |         set_param([gcb '/Verre_int'], 'lambda', '1.2')
      |         set_param([gcb '/Verre_int'], 'e', num2str(evi))
      |         set_param([gcb '/Verre'], 'lambda', infini)
      |         set_param([gcb '/Verre_ext'], 'lambda', '1.2')
      |         set_param([gcb '/Verre_ext'], 'e', num2str(eve))
      |         set_param([gcb '/Gaz_int'], 'heat_tr_coeff', calcul_conv_gaz(sgaz, num2str(eg), sitr, Materiau))
      |         set_param([gcb '/Gaz_ext'], 'heat_tr_coeff', infini)
      |         
      |     case 3
      |         set_param([gcb '/Verre_int'], 'lambda', '1.2')
      |         set_param([gcb '/Verre_int'], 'e', num2str(evi))
      |         set_param([gcb '/Verre'], 'lambda', '1.2')
      |         set_param([gcb '/Verre'], 'e', num2str(ev0))
      |         set_param([gcb '/Verre_ext'], 'lambda', '1.2')
      |         set_param([gcb '/Verre_ext'], 'e', num2str(eve))
      |         set_param([gcb '/Gaz_int'], 'heat_tr_coeff', calcul_conv_gaz(sgaz, num2str(egi), sitr, Materiau))
      |         set_param([gcb '/Gaz_ext'], 'heat_tr_coeff', calcul_conv_gaz(sgaz, num2str(ege), sitr, Materiau))
      | end
      mask TypeOptions typ: Simple | Double | Triple
      mask Callback typ:
      | CaractMateriaux;
      | typ = get_param(gcb, 'typ');
      | gaz = get_param(gcb, 'gaz');
      | itr = get_param(gcb, 'itr');
      | switch typ
      |     case 'Simple'
      |         set_param(gcb, 'MaskVisibilities',{'on';'off';'on';'on';'on';'off';'off';'off';'off';'off';'off';'on';'on';'on'})
      | 
      |     case 'Double'
      |         set_param(gcb, 'MaskVisibilities',{'on';'on';'on';'on';'off';'on';'on';'off';'off';'off';'on';'on';'on';'on'})
      | 
      |     case 'Triple'
      |         set_param(gcb, 'MaskVisibilities',{'on';'on';'on';'on';'off';'on';'off';'on';'on';'on';'on';'on';'on';'on'})
      | end
      | calcul_resistance(gcb, Materiau)
      mask TypeOptions gaz: Air | Argon
      mask Callback gaz: calcul_resistance(gcb, Materiau)
      mask Callback itr: calcul_resistance(gcb, Materiau)
      mask Callback ev:
      | if strcmp(typ, 'Simple')
      |     calcul_resistance(gcb, Materiau)
      | end
      mask Callback evi:
      | if not(strcmp(typ, 'Simple'))
      |     calcul_resistance(gcb, Materiau)
      | end
      mask Callback eg:
      | if strcmp(typ, 'Double')
      |     calcul_resistance(gcb, Materiau)
      | end
      mask Callback egi:
      | if strcmp(typ, 'Triple')
      |     calcul_resistance(gcb, Materiau)
      | end
      mask Callback ev0:
      | if strcmp(typ, 'Triple')
      |     calcul_resistance(gcb, Materiau)
      | end
      mask Callback ege:
      | if strcmp(typ, 'Triple')
      |     calcul_resistance(gcb, Materiau)
      | end
      mask Callback eve:
      | if not(strcmp(typ, 'Simple'))
      |     calcul_resistance(gcb, Materiau)
      | end
      mask Display:
      | CaractMateriaux;
      | image(imread(['Thermique/' Vitrage(get_param(gcb, 'typ')).Image]), [0.2, 0, 0.6, 0.85]);
      | port_label('lconn', 1, 'Int');
      | port_label('rconn', 1, 'Ext');
      | port_label('output', 1, 'T1');
      | port_label('output', 2, 'T2');
      | 
      | 
      | text(0.5,0.95, get_param(gcb, 'typ'), ...
      |      'HorizontalAlignment','center');

== system Library_SII_2018/Automatisme/Vérin ==
  S : Inport
  Constant : Constant  Value=T
  Constant1 : Constant  Value=N
  Vérin A : Stateflow chart  InitFcn=coder.extrinsic('tic')  TreatAsAtomicUnit=on
  r : Outport
  s : Outport  Port=2
  x : Outport  Port=3
  wires:
  Constant1/1 -> Vérin A/3(N)
  Vérin A/3(x) -> x/1
  Constant/1 -> Vérin A/2(T)
  Vérin A/1(r) -> r/1
  Vérin A/2(s) -> s/1
  S/1 -> Vérin A/1(S)
